simulink model "BASK"  (R2018a)
settings: Solver=VariableStepAuto  StartTime=0.0  StopTime=10  RelTol=1e-3
libraries: dspmathops x2, dspsrcs4 x2, commrandsrc3 x1, dspfdesign x1
settings Model: Creator=Souhardhya Paul  LastModifiedBy=Souhardhya Paul

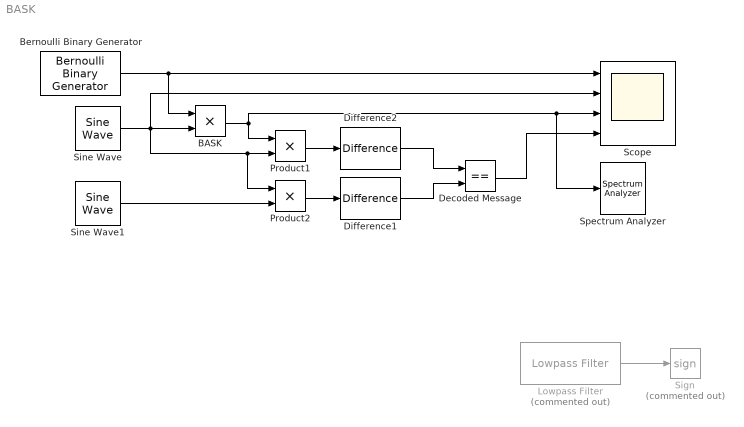
== system BASK ==
  BASK : Product
  Bernoulli Binary Generator : commrandsrc3/Bernoulli Binary Generator  ProbabilityOfZero=0.5  SeedSource=Auto  Seed=0  SampleTime=0.1  SamplesPerFrame=1  OutputDataType=double  SimulateUsing=Interpreted execution
  Decoded Message : RelationalOperator  Operator===  OutDataTypeStr=boolean  RndMeth=Simplest
  Difference1 : dspmathops/Difference  Run=Yes  dim=Columns  Dimension=1  roundingMode=Floor  overflowMode=off  outputDataTypeStr=Inherit: Same as accumulator  outputMin=[]  outputMax=[]  outputLastDataTypeStr=Inherit: Same as accumulator
      settings: SourceProductName=DSP System Toolbox  SourceProductBaseCode=DS
  Difference2 : dspmathops/Difference  Run=Yes  dim=Columns  Dimension=1  roundingMode=Floor  overflowMode=off  outputDataTypeStr=Inherit: Same as accumulator  outputMin=[]  outputMax=[]  outputLastDataTypeStr=Inherit: Same as accumulator
      settings: SourceProductName=DSP System Toolbox  SourceProductBaseCode=DS
  Lowpass Filter : dspfdesign/Lowpass Filter  Commented=on  FilterType=FIR  DesignForMinimumOrder=on  FilterOrder=50  PassbandFrequency=10  StopbandFrequency=80  PassbandRipple=1  StopbandAttenuation=60  InheritSampleRate=on  SampleRate=100  SimulateUsing=Interpreted execution  roundingMode=Floor  coeffsDataTypeStr=fixdt(1,16)
  Product1 : Product
  Product2 : Product
  Scope : Scope  NumInputPorts=4
  Sign : Signum  Commented=on
  Sine Wave : dspsrcs4/Sine Wave  Amplitude=1  Frequency=100  Phase=0  SampleMode=Discrete  OutComplex=Real  CompMethod=Trigonometric fcn  TableSize=Speed  SampleTime=1/1000  SamplesPerFrame=1  ResetState=Restart at time zero  OutputFrames=off  dataType=double  wordLen=16  udDataType=sfix(16)  fracBitsMode=Best precision  numFracBits=15  OutDataTypeStr=double  LastOutDataTypeStr=double
  Sine Wave1 : dspsrcs4/Sine Wave  Amplitude=1  Frequency=100  Phase=0  SampleMode=Discrete  OutComplex=Real  CompMethod=Trigonometric fcn  TableSize=Speed  SampleTime=1/1000  SamplesPerFrame=1  ResetState=Restart at time zero  OutputFrames=off  dataType=double  wordLen=16  udDataType=sfix(16)  fracBitsMode=Best precision  numFracBits=15  OutDataTypeStr=double  LastOutDataTypeStr=double
  Spectrum Analyzer : SpectrumAnalyzer
  wires:
  Bernoulli Binary Generator/1 -> BASK/1, Scope/1
  BASK/1 -> Product1/1, Spectrum Analyzer/1, Scope/3
  Sine Wave/1 -> Product2/1, Product1/2, Scope/2, BASK/2
  Lowpass Filter/1 -> Sign/1
  Product1/1 -> Difference2/1
  Sine Wave1/1 -> Product2/2
  Product2/1 -> Difference1/1
  Difference1/1 -> Decoded Message/2
  Difference2/1 -> Decoded Message/1
  Decoded Message/1 -> Scope/4
